simulink model "RVC_Cartesian_PD_control_gravity_compensation"  (R2020b)
settings: Solver=VariableStepAuto  StartTime=0.0  StopTime=30  RelTol=1e-3
values from neighbouring files (symbols this model uses):
  dotxd = [0 0 0 0 0 0]'    [RVC_main.m]
  gravity = [0 0 9.81]'    [RVC_main.m]
  KD_O = diag([0.1 0.1 0.1 0.005 0.005 0.005])    [RVC_main.m]
  KP_O = diag([0.12 0.12 0.12 0.01 0.01 0.01])    [RVC_main.m]
  xd = kinematics(dh, qd)    [RVC_main.m]    (also in forward_dynamics.m = [x(n+1:2*n); q_ddot])
undefined symbols (not defined in the file or in its folder): Analytical_Jacobian, dh, inv_dyn_recursive_NewtonEulero, kinematics, singularity_alert
libraries: vrlib x1
settings Model: Creator=eros  LastModifiedBy=nicol
settings ExplorerConfigSet: InternalSimMechanicsExplorerSettings="<ExplorerConfiguration><canonicalview>default</canonicalview><AnimationSetting><BasePlaybackSpeed>1.0</BasePlaybackSpeed><PlaybackSpeedFactor>1.0</PlaybackSpeedFactor></AnimationSetting><TilePanel><TileInfo><Tiles Columns=\"1\" Count=\"1\" Rows=\"1\"><Column Weight=\"1\"/><Row Weight=\"1\"/><Tile Height=\"1\" Width=\"1\" X=\"0\" Y=\"0\"/></Tiles></TileInfo><SceneInfo><SceneViewer><BGColor><R>0.60000002384185791</R><G>0.60000002384185791</G><B>0.60000002384185791</B></BGColor><Camera><DoPerspective>off</DoPerspective><Position><X>-0.181684881448745728</X><Y>-0.95036005973815918</Y><Z>-0.22997195273637705</Z></Position><Center><X>-0.181684881448745728</X><Y>0.0496399402618408203</Y><Z>-0.22997195273637705</Z></Center><Up><X>0</X><Y>-0</Y><Z>1</Z></Up><ViewLimDist>1</ViewLimDist><YLim>0.399270979762077316</YLim><XLim>0.625019128657091527</XLim></Camera></SceneViewer></SceneInfo></TilePanel><MechEditorPanel><Cameras/><GfxPanelCameraMap/><VideoCreator><PlaybackSpeedRatio>1.0</PlaybackSpeedRatio><FrameRate>30</FrameRate><VideoFormat>Motion JPEG AVI</VideoFormat><FrameSize>auto</FrameSize></VideoCreator></MechEditorPanel></ExplorerConfiguration>"

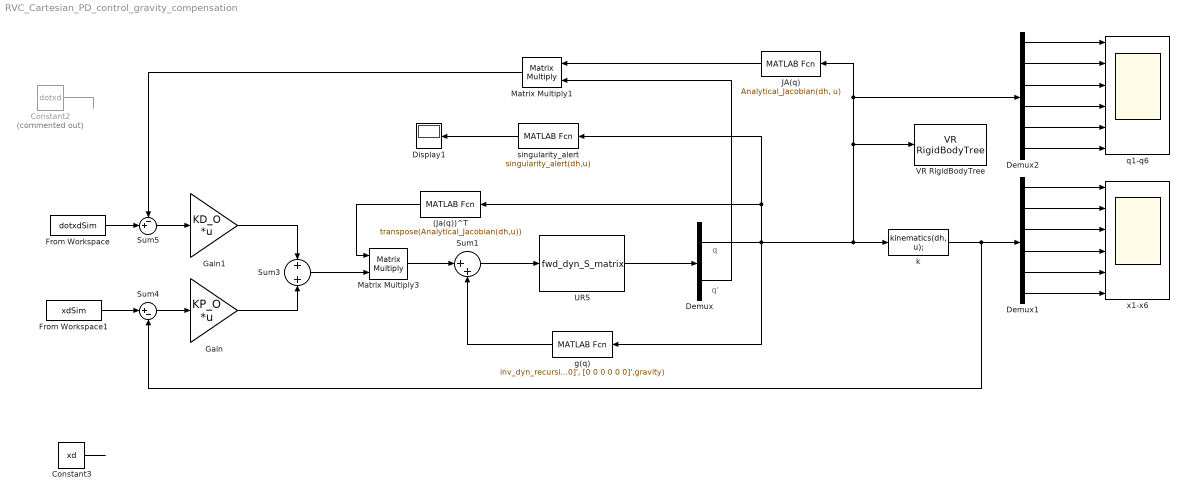
== system RVC_Cartesian_PD_control_gravity_compensation ==
  note: q'
  note: q
  (Ja(q))^T : MATLABFcn  MATLABFcn=transpose(Analytical_Jacobian(dh,u))  OutputDimensions=[dh.dof dh.dof]  Output1D=off
  Constant2 : Constant  Commented=on  Value=dotxd
  Constant3 : Constant  Value=xd
  Demux : Demux  Outputs=2
  Demux1 : Demux  Outputs=dh.dof
  Demux2 : Demux  Outputs=dh.dof
  Display1 : Display
  From Workspace : FromWorkspace  VariableName=dotxdSim
  From Workspace1 : FromWorkspace  VariableName=xdSim
  Gain : Gain  Gain=KP_O  Multiplication=Matrix(K*u)
  Gain1 : Gain  Gain=KD_O  Multiplication=Matrix(K*u)
  JA(q) : MATLABFcn  MATLABFcn=Analytical_Jacobian(dh, u)  OutputDimensions=[dh.dof dh.dof]  Output1D=off
  Matrix Multiply1 : Product  Multiplication=Matrix(*)
  Matrix Multiply3 : Product  Multiplication=Matrix(*)
  Sum1 : Sum  Inputs=|++
  Sum3 : Sum
  Sum4 : Sum  Inputs=|+-
  Sum5 : Sum  Inputs=-+|
  UR5 : S-Function  FunctionName=fwd_dyn_S_matrix  Parameters=dh, he, gravity, q0, dotq0  SFunctionDeploymentMode=off  EnableBusSupport=off
  VR RigidBodyTree : vrlib/VR RigidBodyTree  RBT=UR5_robot  useRBT=on  Ts=-1  ForceViewerOpen=on
      settings: SourceProductBaseCode=SL
  g(q) : MATLABFcn  MATLABFcn=inv_dyn_recursive_NewtonEulero(dh,u,[0 0 0 0 0 0]', [0 0 0 0 0 0]',gravity)  OutputDimensions=[dh.dof 1]  Output1D=off
  k : MATLABFcn  MATLABFcn=kinematics(dh, u);  OutputDimensions=[dh.dof 1]  Output1D=off
  q1-q6 : Scope  NumInputPorts=6
  singularity_alert : MATLABFcn  MATLABFcn=singularity_alert(dh,u)  Output1D=off
  x1-x6 : Scope  NumInputPorts=6
  wires:
  Sum1/1 -> UR5/1
  UR5/1 -> Demux/1
  Sum3/1 -> Matrix Multiply3/2
  (Ja(q))^T/1 -> Matrix Multiply3/1
  singularity_alert/1 -> Display1/1
  Matrix Multiply3/1 -> Sum1/1
  g(q)/1 -> Sum1/2
  Constant2/1 -> ?
  Sum5/1 -> Gain1/1
  Gain/1 -> Sum3/2
  Gain1/1 -> Sum3/1
  Constant3/1 -> ?
  Sum4/1 -> Gain/1
  Matrix Multiply1/1 -> Sum5/1
  JA(q)/1 -> Matrix Multiply1/1
  Demux/2 -> Matrix Multiply1/2
  Demux1/2 -> x1-x6/2
  Demux1/3 -> x1-x6/3
  Demux1/6 -> x1-x6/6
  Demux1/5 -> x1-x6/5
  Demux1/1 -> x1-x6/1
  Demux1/4 -> x1-x6/4
  k/1 -> Demux1/1, Sum4/2
  Demux2/2 -> q1-q6/2
  Demux2/3 -> q1-q6/3
  Demux2/6 -> q1-q6/6
  Demux2/5 -> q1-q6/5
  Demux2/1 -> q1-q6/1
  Demux2/4 -> q1-q6/4
  Demux/1 -> g(q)/1, Demux2/1, JA(q)/1, VR RigidBodyTree/1, k/1, singularity_alert/1, (Ja(q))^T/1
  From Workspace/1 -> Sum5/2
  From Workspace1/1 -> Sum4/1
